simulink model "sampleModel1704"  (R2023a)
settings: Solver=VariableStepAuto  StartTime=0.0  StopTime=10.0  RelTol=1e-3
libraries: hdlsllib x7, simulink x2
settings Model: Creator=user1  LastModifiedBy=user1

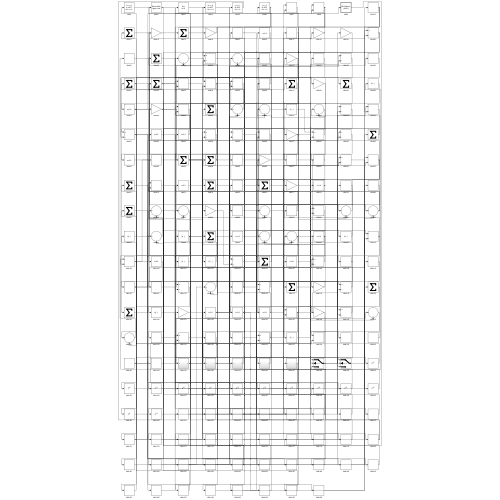
[thumbnail: Simulink's stored preview of the top-level diagram]
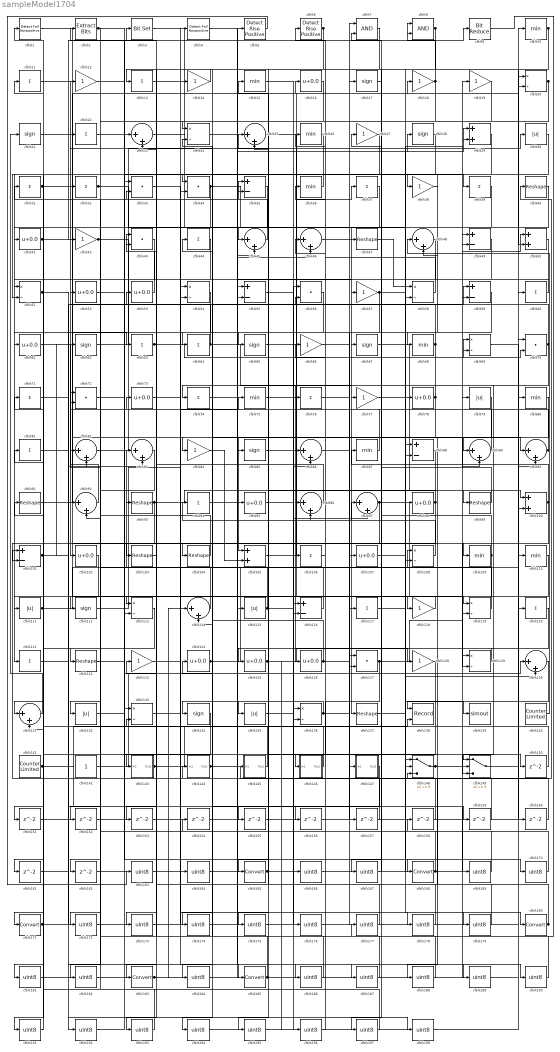
== system sampleModel1704 ==
  cfblk1 : hdlsllib/Logic and Bit Operations/Detect Fall Nonpositive  vinit=0  OutDataTypeStr=boolean
  cfblk{10,15,26,36,68,75,80,87,109..110} (10 alike) : MinMax
  cfblk{29,50,100,105} (4 alike) : Sum
  cfblk{35,49,55,59,88,101,116} (7 alike) : Sum  Inputs=+-
  cfblk{16,41,52..53,61,73,78,95,98,102,107,124..126} (14 alike) : Bias  Bias=0.0  SaturateOnIntegerOverflow=off
  cfblk{40,47,91,93,99,103..104,122,137} (9 alike) : Reshape
  cfblk{11,13,22,31..32,37,39,44,60,63..64,71,74,76,81,94,106,117,120..121} (20 alike) : Sum  Inputs=+
  cfblk{20,24,51,54,58,69,108,113,119,129,133,136} (12 alike) : Product  Inputs=*/  RndMeth=Zero  SaturateOnIntegerOverflow=on
  cfblk{30,79,111,115,132,135} (6 alike) : Abs  SaturateOnIntegerOverflow=off
  cfblk{17,21,28,62,65,67,85,112,134} (9 alike) : Signum
  cfblk{23,25,45..46,48,82..83,86,89..90,92,96..97,114,130..131} (16 alike) : Sum  Inputs=|++
  cfblk{12,14,18..19,27,38,42,57,66,77,84,118,123,128} (14 alike) : Gain
  cfblk{33..34,43,56,70,72,127} (7 alike) : DotProduct  OutDataTypeStr=Inherit: Inherit via internal rule
  cfblk138 : Record  FileSettingsInternal="{\"entries\":[{\"content\":{\"excelSettings\":{\"content\":{},\"type\":\"Streamout.ExcelSettings\"}},\"type\":\"Streamout.FileSettingStorage\",\"uuid\":\"\"}],\"packageUris\":[\"http:\\/\\/schema.mathworks.com\\/mf0\\/streamout_blocks\\/R2020a\"],\"version\":\"1.0\"}"  Layout=[1 1]  SignalsInternal="{\"entries\":[{\"content\":{\"signals\":[{\"content\":{\"blockPath\":[],\"dimensions\":[1],\"domain\":\"\",\"lineColor\":\"#a2142f\",\"plots\":[1],\"port\":1,\"signalID\":3114,\"signalName\":\"XY Graph:1\"},\"type\":\"RecordBlkView.Signal\",\"uuid\":\"\"},{\"content\":{\"blockPath\":[],\"dimensions\":[1],\"domain\":\"\",\"lineColor\":\"#139fff\",\"plots\":[1],\"port\":2,\"signalID\":3117,\"signalName\":\"XY Graph:2\"},\"type\":\"RecordBlkView.Signal\",\"uuid\":\"\"}]},\"type\":\"RecordBlkView.InputSignals\",\"uuid\":\"\"}],\"packageUris\":[\"http:\\/\\/schema.mathworks.com\\/mf0\\/streamout_blocks\\/R2020a\"],\"version\":\"1.0\"}"  VisualizationBindings="{\"xyplotplugin\":{\"info\":[{\"series\":[{\"bindingParametersList\":[{\"parameter\":\"X-Axis\",\"signalID\":3114,\"signalName\":\"XY Graph:1\"},{\"parameter\":\"Y-Axis\",\"signalID\":3117,\"signalName\":\"XY Graph:2\"}],\"seriesID\":791}],\"subplotID\":1}]}}"  CompatibilityTag=XY  st=-1
  cfblk139 : ToWorkspace  VariableName=simout  SaveFormat=Timeseries  SampleTime=-1
  cfblk140 : hdlsllib/Sources/Counter Limited  uplimit=7  tsamp=-1
  cfblk141 : hdlsllib/Sources/Counter Limited  uplimit=7  tsamp=-1
  cfblk142 : Constant  SampleTime=-1
  cfblk143 : Subsystem
      settings: LibrarySourceBlock=|
      | hdlsllib/Ports &
      | Subsystems/Subsystem
  cfblk144 : Subsystem
      settings: LibrarySourceBlock=|
      | hdlsllib/Ports &
      | Subsystems/Subsystem
  cfblk145 : Subsystem
      settings: LibrarySourceBlock=|
      | hdlsllib/Ports &
      | Subsystems/Subsystem
  cfblk146 : Subsystem
      settings: LibrarySourceBlock=|
      | hdlsllib/Ports &
      | Subsystems/Subsystem
  cfblk147 : Subsystem
      settings: LibrarySourceBlock=|
      | hdlsllib/Ports &
      | Subsystems/Subsystem
  cfblk148 : Switch  SaturateOnIntegerOverflow=off  InputSameDT=off
  cfblk149 : Switch  SaturateOnIntegerOverflow=off  InputSameDT=off
  cfblk{150..162} (13 alike) : Delay  SampleTime=1
  cfblk{163..164,166..167,169..170,172..179,181..182,184,186..198} (30 alike) : DataTypeConversion  OutDataTypeStr=uint8  SaturateOnIntegerOverflow=off  RndMeth=Floor
  cfblk{165,168,171,180,183,185} (6 alike) : DataTypeConversion  SaturateOnIntegerOverflow=off  RndMeth=Floor
  cfblk2 : simulink/Logic and Bit Operations/Extract Bits  bitsToExtract=Upper half  numBits=8  bitIdxRange=[0 7]  outScalingMode=Preserve fixed-point scaling
      settings: LibrarySourceBlock=|
      | hdlsllib/Logic and Bit
      | Operations/Extract Bits
  cfblk3 : simulink/Logic and Bit Operations/Bit Set  iBit=0
      settings: LibrarySourceBlock=|
      | hdlsllib/Logic and Bit
      | Operations/Bit Set
  cfblk4 : hdlsllib/Logic and Bit Operations/Detect Fall Nonpositive  vinit=0  OutDataTypeStr=boolean
  cfblk5 : hdlsllib/Logic and Bit Operations/Detect Rise Positive  vinit=0  OutDataTypeStr=boolean
  cfblk6 : hdlsllib/Logic and Bit Operations/Detect Rise Positive  vinit=0  OutDataTypeStr=boolean
  cfblk7 : Logic  AllPortsSameDT=off  OutDataTypeStr=boolean
  cfblk8 : Logic  AllPortsSameDT=off  OutDataTypeStr=boolean
  cfblk9 : hdlsllib/Logic and Bit Operations/Bit Reduce  mode=AND
  wires:
  cfblk105/1 -> cfblk37/1
  cfblk36/1 -> cfblk121/1
  cfblk82/1 -> cfblk84/1
  cfblk101/1 -> cfblk62/1, cfblk189/1
  cfblk146/1(Out1) -> cfblk91/1
  cfblk62/1 -> cfblk30/1
  cfblk140/1 -> cfblk48/1
  cfblk79/1 -> cfblk105/1
  cfblk91/1 -> cfblk16/1
  cfblk130/1 -> cfblk138/1
  cfblk67/1 -> cfblk100/1
  cfblk11/1 -> cfblk119/1
  cfblk114/1 -> cfblk83/1
  cfblk133/1 -> cfblk185/1
  cfblk109/1 -> cfblk73/1, cfblk162/1
  cfblk84/1 -> cfblk105/2
  cfblk46/1 -> cfblk137/1
  cfblk31/1 -> cfblk83/2, cfblk61/1
  cfblk65/1 -> cfblk118/1
  cfblk100/1 -> cfblk87/1, cfblk129/2
  cfblk29/1 -> cfblk68/1
  cfblk144/1(Out1) -> cfblk40/1, cfblk29/2
  cfblk85/1 -> cfblk89/1
  cfblk97/1 -> cfblk129/1, cfblk101/2
  cfblk61/1 -> cfblk102/1
  cfblk41/1 -> cfblk109/1, cfblk111/1, cfblk9/1
  cfblk21/1 -> cfblk89/2
  cfblk4/1 -> cfblk57/1
  cfblk42/1 -> cfblk117/1, cfblk8/2
  cfblk89/1 -> cfblk3/1
  cfblk124/1 -> cfblk20/1, cfblk28/1, cfblk46/2
  cfblk3/1 -> cfblk38/1
  cfblk1/1 -> cfblk63/1
  cfblk127/1 -> cfblk49/1, cfblk146/1(In1)
  cfblk75/1 -> cfblk10/1
  cfblk35/1 -> cfblk45/1
  cfblk47/1 -> cfblk58/1
  cfblk131/1 -> cfblk21/1
  cfblk107/1 -> cfblk58/2
  cfblk111/1 -> cfblk20/2, cfblk59/1
  cfblk93/1 -> cfblk99/1, cfblk75/1, cfblk151/1
  cfblk53/1 -> cfblk43/1
  cfblk60/1 -> cfblk51/1
  cfblk141/1 -> cfblk88/1, cfblk169/1
  cfblk8/1 -> cfblk67/1, cfblk47/1
  cfblk125/1 -> cfblk128/1, cfblk196/1
  cfblk112/1 -> cfblk14/1
  cfblk44/1 -> cfblk112/1
  cfblk87/1 -> cfblk35/1
  cfblk121/1 -> cfblk92/1
  cfblk110/1 -> cfblk183/1
  cfblk2/1 -> cfblk35/2, cfblk182/1
  cfblk103/1 -> cfblk43/2
  cfblk66/1 -> cfblk17/1
  cfblk92/1 -> cfblk12/1
  cfblk90/1 -> cfblk42/1, cfblk46/1
  cfblk63/1 -> cfblk70/2, cfblk106/1, cfblk149/2, cfblk149/3
  cfblk136/1 -> cfblk69/1, cfblk134/1
  cfblk16/1 -> cfblk64/1
  cfblk126/1 -> cfblk22/1, cfblk18/1
  cfblk142/1 -> cfblk119/2
  cfblk33/1 -> cfblk168/1
  cfblk137/1 -> cfblk29/1
  cfblk26/1 -> cfblk51/2
  cfblk78/1 -> cfblk104/1, cfblk76/1
  cfblk86/1 -> cfblk69/2
  cfblk64/1 -> cfblk77/1, cfblk32/1
  cfblk88/1 -> cfblk135/1
  cfblk51/1 -> cfblk156/1, cfblk198/1
  cfblk117/1 -> cfblk139/1
  cfblk24/1 -> cfblk95/1
  cfblk143/1(Out1) -> cfblk138/2, cfblk108/1
  cfblk96/1 -> cfblk2/1
  cfblk115/1 -> cfblk72/1, cfblk86/2
  cfblk54/1 -> cfblk171/1
  cfblk20/1 -> cfblk23/2, cfblk172/1
  cfblk68/1 -> cfblk74/1, cfblk26/1
  cfblk59/1 -> cfblk127/2
  cfblk23/1 -> cfblk78/1
  cfblk13/1 -> cfblk4/1
  cfblk83/1 -> cfblk122/1
  cfblk32/1 -> cfblk145/1(In1), cfblk39/1
  cfblk116/1 -> cfblk25/1
  cfblk99/1 -> cfblk27/1
  cfblk38/1 -> cfblk48/2
  cfblk55/1 -> cfblk180/1
  cfblk25/1 -> cfblk90/1
  cfblk40/1 -> cfblk41/1
  cfblk14/1 -> cfblk13/1
  cfblk104/1 -> cfblk31/1
  cfblk129/1 -> cfblk125/1
  cfblk58/1 -> cfblk6/1
  cfblk113/1 -> cfblk131/1
  cfblk18/1 -> cfblk8/1, cfblk85/1
  cfblk149/1 -> cfblk90/2
  cfblk94/1 -> cfblk115/1
  cfblk10/1 -> cfblk88/2, cfblk50/2, cfblk184/1
  cfblk70/1 -> cfblk126/1, cfblk149/1, cfblk24/2, cfblk108/2
  cfblk135/1 -> cfblk97/2
  cfblk148/1 -> cfblk79/1, cfblk50/1
  cfblk34/1 -> cfblk116/1, cfblk143/1(In1)
  cfblk145/1(Out1) -> cfblk53/1
  cfblk132/1 -> cfblk130/1
  cfblk57/1 -> cfblk130/2, cfblk113/2
  cfblk118/1 -> cfblk113/1
  cfblk27/1 -> cfblk131/2
  cfblk39/1 -> cfblk65/1
  cfblk45/1 -> cfblk11/1
  cfblk108/1 -> cfblk94/1
  cfblk12/1 -> cfblk34/1
  cfblk98/1 -> cfblk96/1, cfblk96/2, cfblk103/1
  cfblk48/1 -> cfblk114/2
  cfblk49/1 -> cfblk148/2
  cfblk7/1 -> cfblk165/1
  cfblk43/1 -> cfblk132/1
  cfblk106/1 -> cfblk66/1
  cfblk6/1 -> cfblk24/1, cfblk173/1
  cfblk119/1 -> cfblk93/1
  cfblk122/1 -> cfblk150/1
  cfblk150/1 -> cfblk1/1
  cfblk151/1 -> cfblk34/2
  cfblk37/1 -> cfblk152/1
  cfblk152/1 -> cfblk45/2
  cfblk50/1 -> cfblk153/1
  cfblk153/1 -> cfblk148/1
  cfblk154/1 -> cfblk127/1
  cfblk72/1 -> cfblk155/1
  cfblk155/1 -> cfblk116/2
  cfblk156/1 -> cfblk100/2
  cfblk76/1 -> cfblk157/1
  cfblk157/1 -> cfblk101/1
  cfblk158/1 -> cfblk25/2
  cfblk52/1 -> cfblk159/1
  cfblk159/1 -> cfblk97/1
  cfblk69/1 -> cfblk160/1
  cfblk160/1 -> cfblk136/1
  cfblk134/1 -> cfblk161/1
  cfblk162/1 -> cfblk19/1
  cfblk5/1 -> cfblk163/1
  cfblk163/1 -> cfblk107/1
  cfblk73/1 -> cfblk164/1
  cfblk164/1 -> cfblk5/1
  cfblk165/1 -> cfblk86/1, cfblk98/1
  cfblk95/1 -> cfblk166/1
  cfblk166/1 -> cfblk7/1
  cfblk17/1 -> cfblk167/1
  cfblk167/1 -> cfblk7/2
  cfblk168/1 -> cfblk36/1, cfblk92/2
  cfblk169/1 -> cfblk33/1
  cfblk22/1 -> cfblk170/1
  cfblk170/1 -> cfblk33/2
  cfblk171/1 -> cfblk49/2, cfblk82/2
  cfblk172/1 -> cfblk54/1
  cfblk173/1 -> cfblk54/2
  cfblk147/1(Out1) -> cfblk174/1
  cfblk174/1 -> cfblk144/1(In1)
  cfblk19/1 -> cfblk175/1
  cfblk175/1 -> cfblk147/1(In1)
  cfblk15/1 -> cfblk176/1
  cfblk176/1 -> cfblk70/1
  cfblk9/1 -> cfblk177/1
  cfblk177/1 -> cfblk15/1
  cfblk123/1 -> cfblk178/1
  cfblk178/1 -> cfblk154/1
  cfblk77/1 -> cfblk179/1
  cfblk179/1 -> cfblk123/1
  cfblk180/1 -> cfblk158/1, cfblk148/3
  cfblk28/1 -> cfblk181/1
  cfblk181/1 -> cfblk55/1
  cfblk182/1 -> cfblk55/2
  cfblk183/1 -> cfblk59/2, cfblk114/1
  cfblk184/1 -> cfblk110/1
  cfblk185/1 -> cfblk136/2, cfblk52/1, cfblk44/1
  cfblk74/1 -> cfblk186/1
  cfblk186/1 -> cfblk133/1
  cfblk161/1 -> cfblk187/1
  cfblk187/1 -> cfblk133/2
  cfblk80/1 -> cfblk188/1
  cfblk188/1 -> cfblk124/1
  cfblk189/1 -> cfblk80/1
  cfblk71/1 -> cfblk190/1
  cfblk190/1 -> cfblk82/1
  cfblk102/1 -> cfblk191/1
  cfblk191/1 -> cfblk71/1
  cfblk81/1 -> cfblk192/1
  cfblk192/1 -> cfblk23/1
  cfblk30/1 -> cfblk193/1
  cfblk193/1 -> cfblk81/1
  cfblk56/1 -> cfblk194/1
  cfblk194/1 -> cfblk60/1
  cfblk128/1 -> cfblk195/1
  cfblk195/1 -> cfblk56/1
  cfblk196/1 -> cfblk56/2
  cfblk120/1 -> cfblk197/1
  cfblk197/1 -> cfblk72/2
  cfblk198/1 -> cfblk120/1

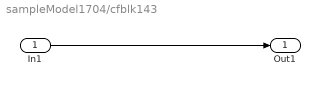
== system sampleModel1704/cfblk143 ==
  In1 : Inport
  Out1 : Outport
  wires:
  In1/1 -> Out1/1

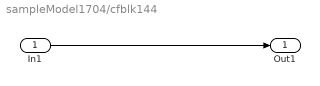
== system sampleModel1704/cfblk144 ==
  In1 : Inport
  Out1 : Outport
  wires:
  In1/1 -> Out1/1

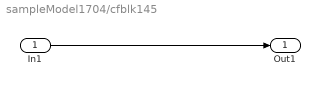
== system sampleModel1704/cfblk145 ==
  In1 : Inport
  Out1 : Outport
  wires:
  In1/1 -> Out1/1

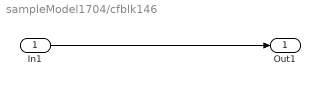
== system sampleModel1704/cfblk146 ==
  In1 : Inport
  Out1 : Outport
  wires:
  In1/1 -> Out1/1

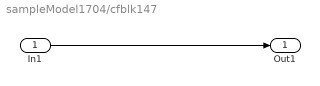
== system sampleModel1704/cfblk147 ==
  In1 : Inport
  Out1 : Outport
  wires:
  In1/1 -> Out1/1
